simulink library "Custom_Library"  (R2023a)
settings: Solver=VariableStepAuto  StartTime=0.0  StopTime=10.0  RelTol=1e-3
values from neighbouring files (symbols this model uses):
  AEP = 0.03    [simulation_setup.m]
  max_torque_alpha = globalTorque    (= 0.94)    [simulation_setup.m]
  max_torque_beta = globalTorque    (= 0.94)    [simulation_setup.m]
  max_torque_gamma = globalTorque    (= 0.94)    [simulation_setup.m]
  N = 16    [rl_setup.m]
  PEP = -0.03    [simulation_setup.m]
  pid_D = 1    [simulation_setup.m]
  pid_filter_N = 1000    [simulation_setup.m]
  pid_I = 0.1    [simulation_setup.m]
  pid_P = 600    [simulation_setup.m]
  step_height = 0.06    [simulation_setup.m]
  step_length = 0.04    [simulation_setup.m]
undefined symbols (not defined in the file or in its folder): X, Y, Z
libraries: sm_lib x31, nesl_utility x13, $bdroot x5, slpidlib x3
(part 2 of 2)

== system Custom_Library/Hexapod Leg/Coxa ==
  Inertia : sm_lib/Body Elements/Inertia  InertiaType=Custom  Mass=0.02471  MassUnits=kg  CenterOfMass=[0, 0, 0]  CenterOfMassUnits=m  MomentsOfInertia=[2.154e-05, 2.657e-05, 2.925e-05]  MomentsOfInertiaUnits=kg*m^2  ProductsOfInertia=[-1.000000000000002e-11, -1.92741e-06, -1.22e-09]  ProductsOfInertiaUnits=kg*m^2  GraphicType=None  MarkerShape=Inertia  MarkerSize=20  GraphicVisPropType=SimpleVisualProperties  GraphicDiffuseColor=[0.5 0.5 0.5]  GraphicSpecularColor=[0.5 0.5 0.5 1.0]  GraphicAmbientColor=[0.15 0.15 0.15 1.0]  GraphicEmissiveColor=[0.0 0.0 0.0 1.0]  GraphicShininess=75  GraphicOpacity=1.0
  InertiaOriginTransform : sm_lib/Frames and Transforms/Rigid Transform  TranslationMethod=Cartesian  TranslationStandardOffset=0  TranslationStandardOffsetUnits=m  TranslationStandardAxis=+Z  TranslationCartesianOffset=[0.019066, -2e-06, 0.006577]  TranslationCartesianOffsetUnits=m  TranslationROffset=0  TranslationROffsetUnits=m  TranslationZOffset=0  TranslationZOffsetUnits=m  TranslationThetaOffset=0  TranslationThetaOffsetUnits=deg  RotationMethod=RotationSequence  RotationAngleUnits=deg  RotationStandardAxis=+Z  RotationAngle=0.0  RotationArbitraryAxis=[0 0 1]  FollAlignAxisA=+X  BaseAlignAxisA=+Y  FollAlignAxisB=+Y  BaseAlignAxisB=+Z  RotationSequenceAxes=BaseAxes  RotationSequence=XYZ  RotationSequenceAngles=[0, 0, 0]  RotationSequenceAnglesUnits=rad  RotationMatrix=[1 0 0; 0 1 0; 0 0 1]  Quaternion=[1 0 0 0]
  ReferenceFrame : sm_lib/Frames and Transforms/Reference Frame
  Spatial Contact Force : sm_lib/Forces and Torques/Spatial Contact Force  SenseContactBaseRotation=off  SenseContactBaseTranslation=off  CoefficientOfDynamicFriction=mu_dynamic  CoefficientOfStaticFriction=mu_static  NormalDamping=damping  NormalDampingUnits=N/(m/s)  SenseContactSignal=off  NormalStiffness=stiffness  NormalStiffnessUnits=N/m  FrictionalCriticalVelocity=critical_vel  FrictionalCriticalVelocityUnits=m/s  ZeroCrossDetectContactStartAndEnd=off  SenseContactFollowerRotation=off  SenseContactFollowerTranslation=off  FrictionType=SmoothStickSlip  SenseFrictionalForceMagnitude=off  SenseNormalForceMagnitude=off  NormalForceType=SmoothSpringDamper  SenseNormalVelocity=off  SenseSeparationDistance=off  SenseTangentialVelocity=off  NormalTransitionRegionWidth=transition_region  NormalTransitionRegionWidthUnits=m
  Visual : sm_lib/Body Elements/File Solid  ExtGeomFileName=C:\Users\basti\OneDrive\Dokumente\Eigene Dokumente\Bachelorarbeit\Bachelor-Thesis\MATLAB\robot_models\interbotix_xshexapod_descriptions\meshes\pxmark4_meshes\pxmark4_coxa_link.stl  UnitType=Custom  ExtGeomFileUnits=mm  StepReaderType=HEX  ExportConvexHullGeometry=on  InertiaType=Custom  Mass=0  MassUnits=kg  CenterOfMass=[0, 0, 0]  CenterOfMassUnits=m  MomentsOfInertia=[0, 0, 0]  MomentsOfInertiaUnits=kg*m^2  ProductsOfInertia=[0, 0, 0]  ProductsOfInertiaUnits=kg*m^2  BasedOnType=DensityFromFile  Density=1000  DensityUnits=kg/m^3  DoExposeReferenceFrame=on  SerializedFrames=<Frames/>  GraphicType=FromGeometry  MarkerShape=Sphere  MarkerSize=10  GraphicVisPropType=SimpleVisualProperties  GraphicDiffuseColor=[0.5, 0.5, 0.5]  GraphicSpecularColor=[0.5 0.5 0.5 1.0]  GraphicAmbientColor=[0.15 0.15 0.15 1.0]  GraphicEmissiveColor=[0.0 0.0 0.0 1.0]  GraphicShininess=75  GraphicOpacity=1
  VisualOriginTransform : sm_lib/Frames and Transforms/Rigid Transform  TranslationMethod=Cartesian  TranslationStandardOffset=0  TranslationStandardOffsetUnits=m  TranslationStandardAxis=+Z  TranslationCartesianOffset=[0, 0, 0]  TranslationCartesianOffsetUnits=m  TranslationROffset=0  TranslationROffsetUnits=m  TranslationZOffset=0  TranslationZOffsetUnits=m  TranslationThetaOffset=0  TranslationThetaOffsetUnits=deg  RotationMethod=RotationSequence  RotationAngleUnits=deg  RotationStandardAxis=+Z  RotationAngle=0.0  RotationArbitraryAxis=[0 0 1]  FollAlignAxisA=+X  BaseAlignAxisA=+Y  FollAlignAxisB=+Y  BaseAlignAxisB=+Z  RotationSequenceAxes=BaseAxes  RotationSequence=XYZ  RotationSequenceAngles=[0, 0, 0]  RotationSequenceAnglesUnits=rad  RotationMatrix=[1 0 0; 0 1 0; 0 0 1]  Quaternion=[1 0 0 0]
  left_front_coxa_AxisInvTransform : sm_lib/Frames and Transforms/Rigid Transform  TranslationMethod=Cartesian  TranslationStandardOffset=0  TranslationStandardOffsetUnits=m  TranslationStandardAxis=+Z  TranslationCartesianOffset=[0, 0, 0]  TranslationCartesianOffsetUnits=m  TranslationROffset=0  TranslationROffsetUnits=m  TranslationZOffset=0  TranslationZOffsetUnits=m  TranslationThetaOffset=0  TranslationThetaOffsetUnits=deg  RotationMethod=ArbitraryAxis  RotationAngleUnits=rad  RotationStandardAxis=+Z  RotationAngle=0  RotationArbitraryAxis=[1, 0, 0]  FollAlignAxisA=+X  BaseAlignAxisA=+Y  FollAlignAxisB=+Y  BaseAlignAxisB=+Z  RotationSequenceAxes=FollowerAxes  RotationSequence=XYX  RotationSequenceAngles=[0 0 0]  RotationSequenceAnglesUnits=deg  RotationMatrix=[1 0 0; 0 1 0; 0 0 1]  Quaternion=[1 0 0 0]
  left_front_femur_AxisTransform : sm_lib/Frames and Transforms/Rigid Transform  TranslationMethod=Cartesian  TranslationStandardOffset=0  TranslationStandardOffsetUnits=m  TranslationStandardAxis=+Z  TranslationCartesianOffset=[0, 0, 0]  TranslationCartesianOffsetUnits=m  TranslationROffset=0  TranslationROffsetUnits=m  TranslationZOffset=0  TranslationZOffsetUnits=m  TranslationThetaOffset=0  TranslationThetaOffsetUnits=deg  RotationMethod=ArbitraryAxis  RotationAngleUnits=rad  RotationStandardAxis=+Z  RotationAngle=1.570796326794897  RotationArbitraryAxis=[-1, 0, 0]  FollAlignAxisA=+X  BaseAlignAxisA=+Y  FollAlignAxisB=+Y  BaseAlignAxisB=+Z  RotationSequenceAxes=FollowerAxes  RotationSequence=XYX  RotationSequenceAngles=[0 0 0]  RotationSequenceAnglesUnits=deg  RotationMatrix=[1 0 0; 0 1 0; 0 0 1]  Quaternion=[1 0 0 0]
  left_front_femur_OriginTransform : sm_lib/Frames and Transforms/Rigid Transform  TranslationMethod=Cartesian  TranslationStandardOffset=0  TranslationStandardOffsetUnits=m  TranslationStandardAxis=+Z  TranslationCartesianOffset=[0.052907539, 0, 0]  TranslationCartesianOffsetUnits=m  TranslationROffset=0  TranslationROffsetUnits=m  TranslationZOffset=0  TranslationZOffsetUnits=m  TranslationThetaOffset=0  TranslationThetaOffsetUnits=deg  RotationMethod=RotationSequence  RotationAngleUnits=deg  RotationStandardAxis=+Z  RotationAngle=0.0  RotationArbitraryAxis=[0 0 1]  FollAlignAxisA=+X  BaseAlignAxisA=+Y  FollAlignAxisB=+Y  BaseAlignAxisB=+Z  RotationSequenceAxes=BaseAxes  RotationSequence=XYZ  RotationSequenceAngles=[0, 0, 0]  RotationSequenceAnglesUnits=rad  RotationMatrix=[1 0 0; 0 1 0; 0 0 1]  Quaternion=[1 0 0 0]
  F : PMIOPort  Side=Left
  G : PMIOPort  Port=2  Side=Left
  F1 : PMIOPort  Port=3  Side=Right
  connections:
  Inertia/RConn1 -- InertiaOriginTransform/RConn1
  ReferenceFrame/RConn1 -- InertiaOriginTransform/LConn1 -- left_front_coxa_AxisInvTransform/LConn1 -- left_front_femur_OriginTransform/LConn1 -- VisualOriginTransform/LConn1
  Visual/RConn1 -- VisualOriginTransform/RConn1
  left_front_coxa_AxisInvTransform/RConn1 -- F/RConn1
  left_front_femur_AxisTransform/RConn1 -- F1/RConn1
  left_front_femur_AxisTransform/LConn1 -- left_front_femur_OriginTransform/RConn1
  G/RConn1 -- Spatial Contact Force/LConn1
  Spatial Contact Force/RConn1 -- Visual/LConn1

== system Custom_Library/Hexapod Leg/Femur ==
  Inertia : sm_lib/Body Elements/Inertia  InertiaType=Custom  Mass=0.08583399999999999  MassUnits=kg  CenterOfMass=[0, 0, 0]  CenterOfMassUnits=m  MomentsOfInertia=[2.887e-05, 7.502e-05, 8.672e-05]  MomentsOfInertiaUnits=kg*m^2  ProductsOfInertia=[2.999999999999994e-10, 4.8494e-06, 2.419e-07]  ProductsOfInertiaUnits=kg*m^2  GraphicType=None  MarkerShape=Inertia  MarkerSize=20  GraphicVisPropType=SimpleVisualProperties  GraphicDiffuseColor=[0.5 0.5 0.5]  GraphicSpecularColor=[0.5 0.5 0.5 1.0]  GraphicAmbientColor=[0.15 0.15 0.15 1.0]  GraphicEmissiveColor=[0.0 0.0 0.0 1.0]  GraphicShininess=75  GraphicOpacity=1.0
  InertiaOriginTransform : sm_lib/Frames and Transforms/Rigid Transform  TranslationMethod=Cartesian  TranslationStandardOffset=0  TranslationStandardOffsetUnits=m  TranslationStandardAxis=+Z  TranslationCartesianOffset=[0.020226, -0.00029, -0.00063]  TranslationCartesianOffsetUnits=m  TranslationROffset=0  TranslationROffsetUnits=m  TranslationZOffset=0  TranslationZOffsetUnits=m  TranslationThetaOffset=0  TranslationThetaOffsetUnits=deg  RotationMethod=RotationSequence  RotationAngleUnits=deg  RotationStandardAxis=+Z  RotationAngle=0.0  RotationArbitraryAxis=[0 0 1]  FollAlignAxisA=+X  BaseAlignAxisA=+Y  FollAlignAxisB=+Y  BaseAlignAxisB=+Z  RotationSequenceAxes=BaseAxes  RotationSequence=XYZ  RotationSequenceAngles=[0, 0, 0]  RotationSequenceAnglesUnits=rad  RotationMatrix=[1 0 0; 0 1 0; 0 0 1]  Quaternion=[1 0 0 0]
  ReferenceFrame : sm_lib/Frames and Transforms/Reference Frame
  Spatial Contact Force : sm_lib/Forces and Torques/Spatial Contact Force  SenseContactBaseRotation=off  SenseContactBaseTranslation=off  CoefficientOfDynamicFriction=mu_dynamic  CoefficientOfStaticFriction=mu_static  NormalDamping=damping  NormalDampingUnits=N/(m/s)  SenseContactSignal=off  NormalStiffness=stiffness  NormalStiffnessUnits=N/m  FrictionalCriticalVelocity=critical_vel  FrictionalCriticalVelocityUnits=m/s  ZeroCrossDetectContactStartAndEnd=off  SenseContactFollowerRotation=off  SenseContactFollowerTranslation=off  FrictionType=SmoothStickSlip  SenseFrictionalForceMagnitude=off  SenseNormalForceMagnitude=off  NormalForceType=SmoothSpringDamper  SenseNormalVelocity=off  SenseSeparationDistance=off  SenseTangentialVelocity=off  NormalTransitionRegionWidth=transition_region  NormalTransitionRegionWidthUnits=m
  Visual : sm_lib/Body Elements/File Solid  ExtGeomFileName=C:\Users\basti\OneDrive\Dokumente\Eigene Dokumente\Bachelorarbeit\Bachelor-Thesis\MATLAB\robot_models\interbotix_xshexapod_descriptions\meshes\pxmark4_meshes\pxmark4_femur_link.stl  UnitType=Custom  ExtGeomFileUnits=mm  StepReaderType=HEX  ExportConvexHullGeometry=on  InertiaType=Custom  Mass=0  MassUnits=kg  CenterOfMass=[0, 0, 0]  CenterOfMassUnits=m  MomentsOfInertia=[0, 0, 0]  MomentsOfInertiaUnits=kg*m^2  ProductsOfInertia=[0, 0, 0]  ProductsOfInertiaUnits=kg*m^2  BasedOnType=DensityFromFile  Density=1000  DensityUnits=kg/m^3  DoExposeReferenceFrame=on  SerializedFrames=<Frames/>  GraphicType=FromGeometry  MarkerShape=Sphere  MarkerSize=10  GraphicVisPropType=SimpleVisualProperties  GraphicDiffuseColor=[0.5, 0.5, 0.5]  GraphicSpecularColor=[0.5 0.5 0.5 1.0]  GraphicAmbientColor=[0.15 0.15 0.15 1.0]  GraphicEmissiveColor=[0.0 0.0 0.0 1.0]  GraphicShininess=75  GraphicOpacity=1
  VisualOriginTransform : sm_lib/Frames and Transforms/Rigid Transform  TranslationMethod=Cartesian  TranslationStandardOffset=0  TranslationStandardOffsetUnits=m  TranslationStandardAxis=+Z  TranslationCartesianOffset=[0, 0, 0]  TranslationCartesianOffsetUnits=m  TranslationROffset=0  TranslationROffsetUnits=m  TranslationZOffset=0  TranslationZOffsetUnits=m  TranslationThetaOffset=0  TranslationThetaOffsetUnits=deg  RotationMethod=RotationSequence  RotationAngleUnits=deg  RotationStandardAxis=+Z  RotationAngle=0.0  RotationArbitraryAxis=[0 0 1]  FollAlignAxisA=+X  BaseAlignAxisA=+Y  FollAlignAxisB=+Y  BaseAlignAxisB=+Z  RotationSequenceAxes=BaseAxes  RotationSequence=XYZ  RotationSequenceAngles=[0, 0, 0]  RotationSequenceAnglesUnits=rad  RotationMatrix=[1 0 0; 0 1 0; 0 0 1]  Quaternion=[1 0 0 0]
  left_front_femur_AxisInvTransform : sm_lib/Frames and Transforms/Rigid Transform  TranslationMethod=Cartesian  TranslationStandardOffset=0  TranslationStandardOffsetUnits=m  TranslationStandardAxis=+Z  TranslationCartesianOffset=[0, 0, 0]  TranslationCartesianOffsetUnits=m  TranslationROffset=0  TranslationROffsetUnits=m  TranslationZOffset=0  TranslationZOffsetUnits=m  TranslationThetaOffset=0  TranslationThetaOffsetUnits=deg  RotationMethod=ArbitraryAxis  RotationAngleUnits=rad  RotationStandardAxis=+Z  RotationAngle=1.570796326794897  RotationArbitraryAxis=[-1, 0, 0]  FollAlignAxisA=+X  BaseAlignAxisA=+Y  FollAlignAxisB=+Y  BaseAlignAxisB=+Z  RotationSequenceAxes=FollowerAxes  RotationSequence=XYX  RotationSequenceAngles=[0 0 0]  RotationSequenceAnglesUnits=deg  RotationMatrix=[1 0 0; 0 1 0; 0 0 1]  Quaternion=[1 0 0 0]
  left_front_tibia_AxisTransform : sm_lib/Frames and Transforms/Rigid Transform  TranslationMethod=Cartesian  TranslationStandardOffset=0  TranslationStandardOffsetUnits=m  TranslationStandardAxis=+Z  TranslationCartesianOffset=[0, 0, 0]  TranslationCartesianOffsetUnits=m  TranslationROffset=0  TranslationROffsetUnits=m  TranslationZOffset=0  TranslationZOffsetUnits=m  TranslationThetaOffset=0  TranslationThetaOffsetUnits=deg  RotationMethod=ArbitraryAxis  RotationAngleUnits=rad  RotationStandardAxis=+Z  RotationAngle=1.570796326794897  RotationArbitraryAxis=[-1, 0, 0]  FollAlignAxisA=+X  BaseAlignAxisA=+Y  FollAlignAxisB=+Y  BaseAlignAxisB=+Z  RotationSequenceAxes=FollowerAxes  RotationSequence=XYX  RotationSequenceAngles=[0 0 0]  RotationSequenceAnglesUnits=deg  RotationMatrix=[1 0 0; 0 1 0; 0 0 1]  Quaternion=[1 0 0 0]
  left_front_tibia_OriginTransform : sm_lib/Frames and Transforms/Rigid Transform  TranslationMethod=Cartesian  TranslationStandardOffset=0  TranslationStandardOffsetUnits=m  TranslationStandardAxis=+Z  TranslationCartesianOffset=[0.06, 0, -0.015]  TranslationCartesianOffsetUnits=m  TranslationROffset=0  TranslationROffsetUnits=m  TranslationZOffset=0  TranslationZOffsetUnits=m  TranslationThetaOffset=0  TranslationThetaOffsetUnits=deg  RotationMethod=RotationSequence  RotationAngleUnits=deg  RotationStandardAxis=+Z  RotationAngle=0.0  RotationArbitraryAxis=[0 0 1]  FollAlignAxisA=+X  BaseAlignAxisA=+Y  FollAlignAxisB=+Y  BaseAlignAxisB=+Z  RotationSequenceAxes=BaseAxes  RotationSequence=XYZ  RotationSequenceAngles=[0, 0, 0]  RotationSequenceAnglesUnits=rad  RotationMatrix=[1 0 0; 0 1 0; 0 0 1]  Quaternion=[1 0 0 0]
  F : PMIOPort  Side=Left
  G : PMIOPort  Port=2  Side=Left
  F1 : PMIOPort  Port=3  Side=Right
  connections:
  Inertia/RConn1 -- InertiaOriginTransform/RConn1
  ReferenceFrame/RConn1 -- InertiaOriginTransform/LConn1 -- left_front_femur_AxisInvTransform/LConn1 -- left_front_tibia_OriginTransform/LConn1 -- VisualOriginTransform/LConn1
  Visual/RConn1 -- VisualOriginTransform/RConn1
  left_front_femur_AxisInvTransform/RConn1 -- F/RConn1
  left_front_tibia_AxisTransform/RConn1 -- F1/RConn1
  left_front_tibia_AxisTransform/LConn1 -- left_front_tibia_OriginTransform/RConn1
  Spatial Contact Force/RConn1 -- Visual/LConn1
  G/RConn1 -- Spatial Contact Force/LConn1

== system Custom_Library/Hexapod Leg/Tibia ==
  Inertia : sm_lib/Body Elements/Inertia  InertiaType=Custom  Mass=0.171825  MassUnits=kg  CenterOfMass=[0, 0, 0]  CenterOfMassUnits=m  MomentsOfInertia=[0.0001762, 0.0005158, 0.0003768000000000001]  MomentsOfInertiaUnits=kg*m^2  ProductsOfInertia=[6.181e-07, 0.0001789, -1.4522e-06]  ProductsOfInertiaUnits=kg*m^2  GraphicType=None  MarkerShape=Inertia  MarkerSize=20  GraphicVisPropType=SimpleVisualProperties  GraphicDiffuseColor=[0.5 0.5 0.5]  GraphicSpecularColor=[0.5 0.5 0.5 1.0]  GraphicAmbientColor=[0.15 0.15 0.15 1.0]  GraphicEmissiveColor=[0.0 0.0 0.0 1.0]  GraphicShininess=75  GraphicOpacity=1.0
  InertiaOriginTransform : sm_lib/Frames and Transforms/Rigid Transform  TranslationMethod=Cartesian  TranslationStandardOffset=0  TranslationStandardOffsetUnits=m  TranslationStandardAxis=+Z  TranslationCartesianOffset=[0.036797, 5.4e-05, -0.011991]  TranslationCartesianOffsetUnits=m  TranslationROffset=0  TranslationROffsetUnits=m  TranslationZOffset=0  TranslationZOffsetUnits=m  TranslationThetaOffset=0  TranslationThetaOffsetUnits=deg  RotationMethod=RotationSequence  RotationAngleUnits=deg  RotationStandardAxis=+Z  RotationAngle=0.0  RotationArbitraryAxis=[0 0 1]  FollAlignAxisA=+X  BaseAlignAxisA=+Y  FollAlignAxisB=+Y  BaseAlignAxisB=+Z  RotationSequenceAxes=BaseAxes  RotationSequence=XYZ  RotationSequenceAngles=[0, 0, 0]  RotationSequenceAnglesUnits=rad  RotationMatrix=[1 0 0; 0 1 0; 0 0 1]  Quaternion=[1 0 0 0]
  ReferenceFrame : sm_lib/Frames and Transforms/Reference Frame
  Spatial Contact Force : sm_lib/Forces and Torques/Spatial Contact Force  SenseContactBaseRotation=off  SenseContactBaseTranslation=off  CoefficientOfDynamicFriction=mu_dynamic  CoefficientOfStaticFriction=mu_static  NormalDamping=damping  NormalDampingUnits=N/(m/s)  SenseContactSignal=off  NormalStiffness=stiffness  NormalStiffnessUnits=N/m  FrictionalCriticalVelocity=critical_vel  FrictionalCriticalVelocityUnits=m/s  ZeroCrossDetectContactStartAndEnd=off  SenseContactFollowerRotation=off  SenseContactFollowerTranslation=off  FrictionType=SmoothStickSlip  SenseFrictionalForceMagnitude=off  SenseNormalForceMagnitude=off  NormalForceType=SmoothSpringDamper  SenseNormalVelocity=off  SenseSeparationDistance=off  SenseTangentialVelocity=off  NormalTransitionRegionWidth=transition_region  NormalTransitionRegionWidthUnits=m
  Visual : sm_lib/Body Elements/File Solid  ExtGeomFileName=C:\Users\basti\OneDrive\Dokumente\Eigene Dokumente\Bachelorarbeit\Bachelor-Thesis\MATLAB\robot_models\interbotix_xshexapod_descriptions\meshes\pxmark4_meshes\pxmark4_tibia_link.stl  UnitType=Custom  ExtGeomFileUnits=mm  StepReaderType=HEX  ExportConvexHullGeometry=on  InertiaType=Custom  Mass=0  MassUnits=kg  CenterOfMass=[0, 0, 0]  CenterOfMassUnits=m  MomentsOfInertia=[0, 0, 0]  MomentsOfInertiaUnits=kg*m^2  ProductsOfInertia=[0, 0, 0]  ProductsOfInertiaUnits=kg*m^2  BasedOnType=DensityFromFile  Density=1000  DensityUnits=kg/m^3  DoExposeReferenceFrame=on  SerializedFrames=<Frames/>  GraphicType=FromGeometry  MarkerShape=Sphere  MarkerSize=10  GraphicVisPropType=SimpleVisualProperties  GraphicDiffuseColor=[0.5, 0.5, 0.5]  GraphicSpecularColor=[0.5 0.5 0.5 1.0]  GraphicAmbientColor=[0.15 0.15 0.15 1.0]  GraphicEmissiveColor=[0.0 0.0 0.0 1.0]  GraphicShininess=75  GraphicOpacity=1
  VisualOriginTransform : sm_lib/Frames and Transforms/Rigid Transform  TranslationMethod=Cartesian  TranslationStandardOffset=0  TranslationStandardOffsetUnits=m  TranslationStandardAxis=+Z  TranslationCartesianOffset=[0, 0, 0]  TranslationCartesianOffsetUnits=m  TranslationROffset=0  TranslationROffsetUnits=m  TranslationZOffset=0  TranslationZOffsetUnits=m  TranslationThetaOffset=0  TranslationThetaOffsetUnits=deg  RotationMethod=RotationSequence  RotationAngleUnits=deg  RotationStandardAxis=+Z  RotationAngle=0.0  RotationArbitraryAxis=[0 0 1]  FollAlignAxisA=+X  BaseAlignAxisA=+Y  FollAlignAxisB=+Y  BaseAlignAxisB=+Z  RotationSequenceAxes=BaseAxes  RotationSequence=XYZ  RotationSequenceAngles=[0, 0, 0]  RotationSequenceAnglesUnits=rad  RotationMatrix=[1 0 0; 0 1 0; 0 0 1]  Quaternion=[1 0 0 0]
  left_front_foot_OriginTransform : sm_lib/Frames and Transforms/Rigid Transform  TranslationMethod=Cartesian  TranslationStandardOffset=0  TranslationStandardOffsetUnits=m  TranslationStandardAxis=+Z  TranslationCartesianOffset=[0.095, 0, -0.09]  TranslationCartesianOffsetUnits=m  TranslationROffset=0  TranslationROffsetUnits=m  TranslationZOffset=0  TranslationZOffsetUnits=m  TranslationThetaOffset=0  TranslationThetaOffsetUnits=deg  RotationMethod=RotationSequence  RotationAngleUnits=deg  RotationStandardAxis=+Z  RotationAngle=0.0  RotationArbitraryAxis=[0 0 1]  FollAlignAxisA=+X  BaseAlignAxisA=+Y  FollAlignAxisB=+Y  BaseAlignAxisB=+Z  RotationSequenceAxes=BaseAxes  RotationSequence=XYZ  RotationSequenceAngles=[0, 0, 0]  RotationSequenceAnglesUnits=rad  RotationMatrix=[1 0 0; 0 1 0; 0 0 1]  Quaternion=[1 0 0 0]
  left_front_tibia_AxisInvTransform : sm_lib/Frames and Transforms/Rigid Transform  TranslationMethod=Cartesian  TranslationStandardOffset=0  TranslationStandardOffsetUnits=m  TranslationStandardAxis=+Z  TranslationCartesianOffset=[0, 0, 0]  TranslationCartesianOffsetUnits=m  TranslationROffset=0  TranslationROffsetUnits=m  TranslationZOffset=0  TranslationZOffsetUnits=m  TranslationThetaOffset=0  TranslationThetaOffsetUnits=deg  RotationMethod=ArbitraryAxis  RotationAngleUnits=rad  RotationStandardAxis=+Z  RotationAngle=1.570796326794897  RotationArbitraryAxis=[-1, 0, 0]  FollAlignAxisA=+X  BaseAlignAxisA=+Y  FollAlignAxisB=+Y  BaseAlignAxisB=+Z  RotationSequenceAxes=FollowerAxes  RotationSequence=XYX  RotationSequenceAngles=[0 0 0]  RotationSequenceAnglesUnits=deg  RotationMatrix=[1 0 0; 0 1 0; 0 0 1]  Quaternion=[1 0 0 0]
  F : PMIOPort  Side=Left
  G : PMIOPort  Port=2  Side=Left
  F1 : PMIOPort  Port=3  Side=Right
  connections:
  Inertia/RConn1 -- InertiaOriginTransform/RConn1
  ReferenceFrame/RConn1 -- InertiaOriginTransform/LConn1 -- left_front_foot_OriginTransform/LConn1 -- left_front_tibia_AxisInvTransform/LConn1 -- VisualOriginTransform/LConn1
  Visual/RConn1 -- VisualOriginTransform/RConn1
  left_front_foot_OriginTransform/RConn1 -- F1/RConn1
  left_front_tibia_AxisInvTransform/RConn1 -- F/RConn1
  Spatial Contact Force/RConn1 -- Visual/LConn1
  G/RConn1 -- Spatial Contact Force/LConn1

== system Custom_Library/Hexapod Leg/Torque Limiting ==
  Input : Inport
  Alpha Limit : Saturate  UpperLimit=max_torque_alpha  LowerLimit=-max_torque_alpha
  Beta Limit : Saturate  UpperLimit=max_torque_beta  LowerLimit=-max_torque_beta
  Bus Selector1 : BusSelector  OutputSignals=torque_alpha,torque_beta,torque_gamma
  Gamma Limit : Saturate  UpperLimit=max_torque_gamma  LowerLimit=-max_torque_gamma
  Alpha : Outport
  Beta : Outport  Port=2
  Gamma : Outport  Port=3
  wires:
  Bus Selector1/1 -> Alpha Limit/1  "<torque_alpha>"
  Input/1 -> Bus Selector1/1
  Bus Selector1/3 -> Gamma Limit/1  "<torque_gamma>"
  Bus Selector1/2 -> Beta Limit/1  "<torque_beta>"
  Alpha Limit/1 -> Alpha/1
  Beta Limit/1 -> Beta/1
  Gamma Limit/1 -> Gamma/1

== system Custom_Library/Signal Generator Linear X (Gen. 2)/Stance Phase ==
  Frequency : Inport
  Reset : ResetPort  DisableCoverage=on
  Add : Sum
  Constant1 : Constant  Value=x_amplitude
  Constant2 : Constant  Value=0
  Constant5 : Constant  Value=x_amplitude
  Constant6 : Constant
  Gain1 : Gain  Gain=-4
  Integrator1 : Integrator
  Product2 : Product
  Product3 : Product
  Saturation : Saturate  UpperLimit=step_length  LowerLimit=-step_length
  X : Outport
  "Z " : Outport  Port=2
  wires:
  Constant2/1 -> "Z "/1
  Constant5/1 -> Add/1
  Constant6/1 -> Integrator1/1
  Add/1 -> Saturation/1
  Product3/1 -> Add/2
  Integrator1/1 -> Product3/2
  Frequency/1 -> Product2/2
  Gain1/1 -> Product2/1
  Product2/1 -> Product3/1
  Saturation/1 -> X/1
  Constant1/1 -> Gain1/1

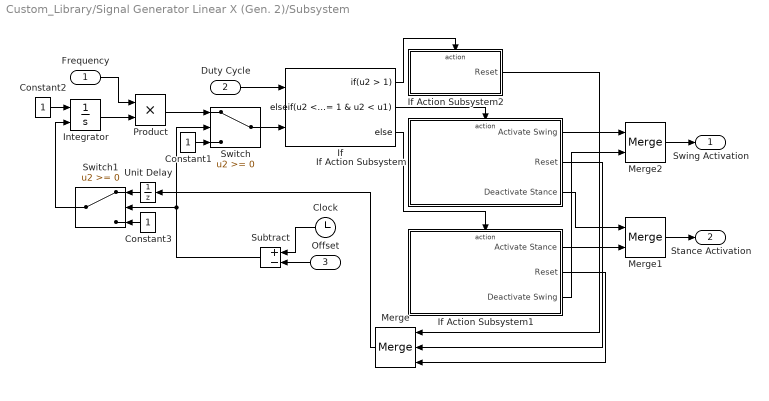
== system Custom_Library/Signal Generator Linear X (Gen. 2)/Subsystem ==
  Frequency : Inport
  Duty Cycle : Inport  Port=2
  Offset : Inport  Port=3
  Clock : Clock
  Constant1 : Constant
  Constant2 : Constant
  Constant3 : Constant
  If : If  NumInputs=2  IfExpression=u2 > 1  ElseIfExpressions=u2 <= 1 & u2 < u1
  If Action Subsystem : Subsystem  TreatAsAtomicUnit=on
  If Action Subsystem1 : Subsystem  TreatAsAtomicUnit=on
  If Action Subsystem2 : Subsystem  TreatAsAtomicUnit=on
  Integrator : Integrator  ExternalReset=level
  Merge : Merge  Inputs=3
  Merge1 : Merge
  Merge2 : Merge
  Product : Product
  Subtract : Sum  Inputs=+-
  Switch : Switch  SaturateOnIntegerOverflow=off  InputSameDT=off
  Switch1 : Switch  SaturateOnIntegerOverflow=off  InputSameDT=off
  Unit Delay : UnitDelay  SampleTime=-1  HasFrameUpgradeWarning=on
  Swing Activation : Outport
  Stance Activation : Outport  Port=2
  wires:
  If Action Subsystem/3(Deactivate Stance) -> Merge1/1
  If/2 -> If Action Subsystem/Action
  Duty Cycle/1 -> If/1
  If/1 -> If Action Subsystem2/Action
  If Action Subsystem1/1(Activate Stance) -> Merge1/2
  If Action Subsystem/2(Reset) -> Merge/2
  Merge/1 -> Unit Delay/1
  If Action Subsystem1/3(Deactivate Swing) -> Merge2/2
  If Action Subsystem2/1(Reset) -> Merge/1
  If Action Subsystem/1(Activate Swing) -> Merge2/1
  If Action Subsystem1/2(Reset) -> Merge/3
  If/3 -> If Action Subsystem1/Action
  Merge2/1 -> Swing Activation/1
  Merge1/1 -> Stance Activation/1
  Switch/1 -> If/2
  Constant1/1 -> Switch/3
  Subtract/1 -> Switch1/2, Switch/2
  Offset/1 -> Subtract/2
  Clock/1 -> Subtract/1
  Integrator/1 -> Product/2
  Product/1 -> Switch/1
  Frequency/1 -> Product/1
  Constant2/1 -> Integrator/1
  Unit Delay/1 -> Switch1/1
  Constant3/1 -> Switch1/3
  Switch1/1 -> Integrator/2

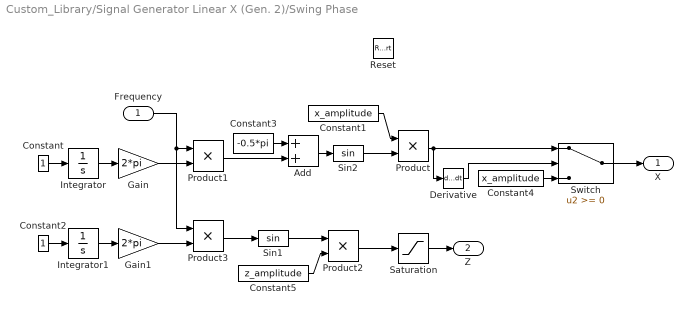
== system Custom_Library/Signal Generator Linear X (Gen. 2)/Swing Phase ==
  Frequency : Inport
  Reset : ResetPort  DisableCoverage=on
  Add : Sum
  Constant : Constant
  Constant1 : Constant  Value=x_amplitude
  Constant2 : Constant
  Constant3 : Constant  Value=-0.5*pi
  Constant4 : Constant  Value=x_amplitude
  Constant5 : Constant  Value=z_amplitude
  Derivative : Derivative
  Gain : Gain  Gain=2*pi
  Gain1 : Gain  Gain=2*pi
  Integrator : Integrator
  Integrator1 : Integrator
  Product{,1..3} (4 alike) : Product
  Saturation : Saturate  UpperLimit=step_height  LowerLimit=0
  Sin1 : Trigonometry
  Sin2 : Trigonometry
  Switch : Switch  SaturateOnIntegerOverflow=off  InputSameDT=off
  X : Outport
  "Z " : Outport  Port=2
  wires:
  Integrator/1 -> Gain/1
  Constant/1 -> Integrator/1
  Sin2/1 -> Product/2
  Constant1/1 -> Product/1
  Product2/1 -> Saturation/1
  Gain/1 -> Product1/2
  Add/1 -> Sin2/1
  Product1/1 -> Add/2
  Constant3/1 -> Add/1
  Product/1 -> Switch/1, Derivative/1
  Constant4/1 -> Switch/3
  Switch/1 -> X/1
  Derivative/1 -> Switch/2
  Product3/1 -> Sin1/1
  Sin1/1 -> Product2/1
  Constant5/1 -> Product2/2
  Constant2/1 -> Integrator1/1
  Gain1/1 -> Product3/2
  Integrator1/1 -> Gain1/1
  Frequency/1 -> Product3/1, Product1/1
  Saturation/1 -> "Z "/1

== system Custom_Library/Signal Generator(Gen. 2)/Stance Phase ==
  Frequency : Inport
  Reset : ResetPort  DisableCoverage=on
  Add : Sum
  Constant : Constant
  Constant1 : Constant  Value=step_length
  Constant2 : Constant  Value=0
  Constant3 : Constant  Value=0.5*pi
  Constant4 : Constant  Value=-step_length
  Derivative : Derivative
  Gain : Gain  Gain=2*pi
  Integrator : Integrator
  Product : Product
  Product1 : Product
  Sin : Trigonometry
  Switch : Switch  Criteria=u2 > Threshold  SaturateOnIntegerOverflow=off  InputSameDT=off
  X : Outport
  "Z " : Outport  Port=2
  wires:
  Integrator/1 -> Gain/1
  Constant/1 -> Integrator/1
  Sin/1 -> Product/2
  Constant1/1 -> Product/1
  Constant2/1 -> "Z "/1
  Frequency/1 -> Product1/1
  Gain/1 -> Product1/2
  Add/1 -> Sin/1
  Product1/1 -> Add/2
  Constant3/1 -> Add/1
  Product/1 -> Derivative/1, Switch/3
  Switch/1 -> X/1
  Derivative/1 -> Switch/2
  Constant4/1 -> Switch/1

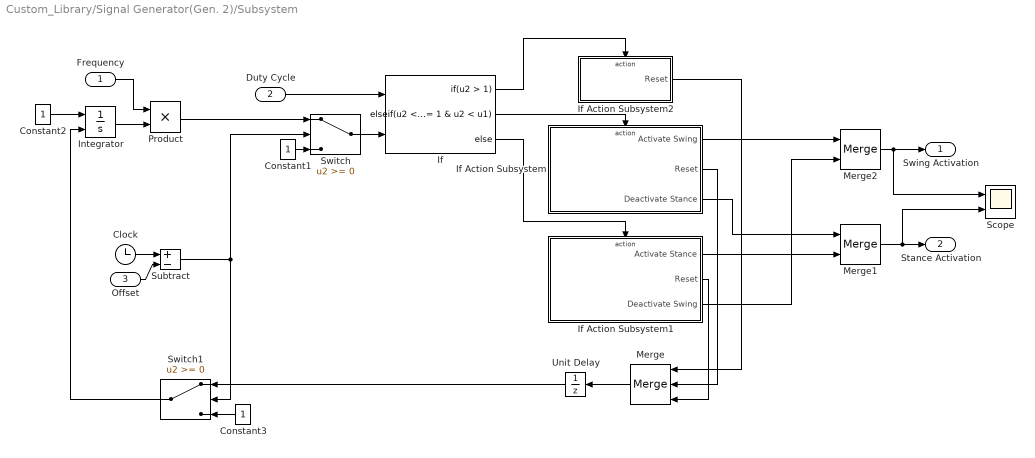
== system Custom_Library/Signal Generator(Gen. 2)/Subsystem ==
  Frequency : Inport
  Duty Cycle : Inport  Port=2
  Offset : Inport  Port=3
  Clock : Clock
  Constant1 : Constant
  Constant2 : Constant
  Constant3 : Constant
  If : If  NumInputs=2  IfExpression=u2 > 1  ElseIfExpressions=u2 <= 1 & u2 < u1
  If Action Subsystem : Subsystem  TreatAsAtomicUnit=on
  If Action Subsystem1 : Subsystem  TreatAsAtomicUnit=on
  If Action Subsystem2 : Subsystem  TreatAsAtomicUnit=on
  Integrator : Integrator  ExternalReset=level
  Merge : Merge  Inputs=3
  Merge1 : Merge
  Merge2 : Merge
  Product : Product
  Scope : Scope  NumInputPorts=2
  Subtract : Sum  Inputs=+-
  Switch : Switch  SaturateOnIntegerOverflow=off  InputSameDT=off
  Switch1 : Switch  SaturateOnIntegerOverflow=off  InputSameDT=off
  Unit Delay : UnitDelay  SampleTime=-1  HasFrameUpgradeWarning=on
  Swing Activation : Outport
  Stance Activation : Outport  Port=2
  wires:
  If Action Subsystem/3(Deactivate Stance) -> Merge1/1
  If/2 -> If Action Subsystem/Action
  Duty Cycle/1 -> If/1
  If/1 -> If Action Subsystem2/Action
  If Action Subsystem1/1(Activate Stance) -> Merge1/2
  If Action Subsystem/2(Reset) -> Merge/2
  Merge/1 -> Unit Delay/1
  If Action Subsystem1/3(Deactivate Swing) -> Merge2/2
  If Action Subsystem2/1(Reset) -> Merge/1
  If Action Subsystem/1(Activate Swing) -> Merge2/1
  If Action Subsystem1/2(Reset) -> Merge/3
  If/3 -> If Action Subsystem1/Action
  Merge2/1 -> Scope/1, Swing Activation/1
  Merge1/1 -> Scope/2, Stance Activation/1
  Switch/1 -> If/2
  Constant1/1 -> Switch/3
  Subtract/1 -> Switch1/2, Switch/2
  Offset/1 -> Subtract/2
  Clock/1 -> Subtract/1
  Integrator/1 -> Product/2
  Product/1 -> Switch/1
  Frequency/1 -> Product/1
  Constant2/1 -> Integrator/1
  Unit Delay/1 -> Switch1/1
  Constant3/1 -> Switch1/3
  Switch1/1 -> Integrator/2

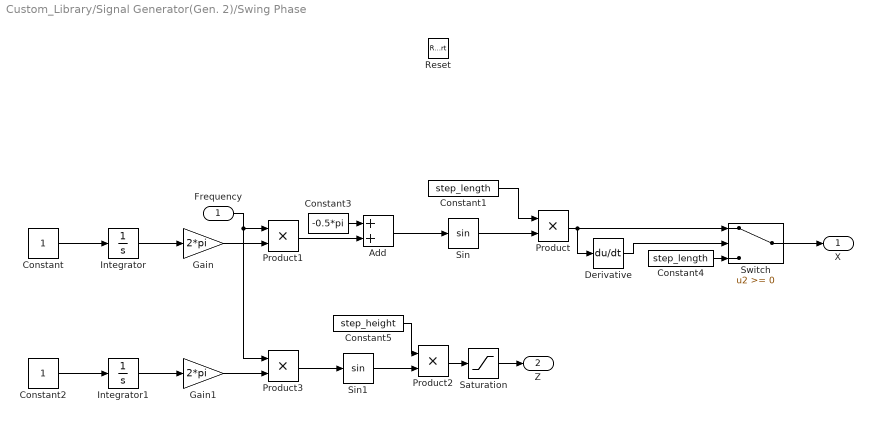
== system Custom_Library/Signal Generator(Gen. 2)/Swing Phase ==
  Frequency : Inport
  Reset : ResetPort  DisableCoverage=on
  Add : Sum
  Constant : Constant
  Constant1 : Constant  Value=step_length
  Constant2 : Constant
  Constant3 : Constant  Value=-0.5*pi
  Constant4 : Constant  Value=step_length
  Constant5 : Constant  Value=step_height
  Derivative : Derivative
  Gain : Gain  Gain=2*pi
  Gain1 : Gain  Gain=2*pi
  Integrator : Integrator
  Integrator1 : Integrator
  Product{,1..3} (4 alike) : Product
  Saturation : Saturate  UpperLimit=step_height  LowerLimit=0
  Sin : Trigonometry
  Sin1 : Trigonometry
  Switch : Switch  SaturateOnIntegerOverflow=off  InputSameDT=off
  X : Outport
  "Z " : Outport  Port=2
  wires:
  Integrator/1 -> Gain/1
  Constant/1 -> Integrator/1
  Sin/1 -> Product/2
  Constant1/1 -> Product/1
  Product2/1 -> Saturation/1
  Gain/1 -> Product1/2
  Add/1 -> Sin/1
  Product1/1 -> Add/2
  Constant3/1 -> Add/1
  Product/1 -> Switch/1, Derivative/1
  Constant4/1 -> Switch/3
  Switch/1 -> X/1
  Derivative/1 -> Switch/2
  Product3/1 -> Sin1/1
  Sin1/1 -> Product2/2
  Constant5/1 -> Product2/1
  Constant2/1 -> Integrator1/1
  Gain1/1 -> Product3/2
  Integrator1/1 -> Gain1/1
  Frequency/1 -> Product3/1, Product1/1
  Saturation/1 -> "Z "/1

== system Custom_Library/Swing-Stance Pattern Generation/Determine Frequencies ==
  note: (1/Hz) *duty_cycle = duty_cycle/Hz = swing_time
      |
      | 1/swing_time = 1 / (duty_cycle/Hz) = Hz/duty_cycle = Hz_for_swing
      | ----------------------------------------------------------------------------------------------------
      | (1/Hz)*(1-duty_cycle) = (1-duty_cycle)/Hz = stance_time
      |
      | 1/stance_time = 1 / ((1-duty_cycle)/Hz) = Hz / (1-duty_cycle) = Hz_for_stance
  Cycle Frequency [Hz] : Inport
  Duty Cycle [%] : Inport  Port=2
  Constant : Constant
  Divide : Product  Inputs=*/
  Divide1 : Product  Inputs=*/
  Subtract : Sum  Inputs=-+
  Swing Frequency [Hz] : Outport
  Stance Frequency [Hz] : Outport  Port=2
  wires:
  Constant/1 -> Subtract/2
  Subtract/1 -> Divide1/2
  Divide1/1 -> Stance Frequency [Hz]/1
  Cycle Frequency [Hz]/1 -> Divide/1, Divide1/1
  Duty Cycle [%]/1 -> Divide/2, Subtract/1
  Divide/1 -> Swing Frequency [Hz]/1

== system Custom_Library/Swing-Stance Pattern Generation/Swing-Stance Signal Generation ==
  note: Initiation of first Swing
      | enables the systems outputs.
      | Prevents stumbling.
  Swing Frequency [Hz] : Inport
  Stance Frequency [Hz] : Inport  Port=2
  Initiate Swing : Inport  Port=3
  Demux : Demux  Outputs=2
  Enable Outputs : Subsystem  TreatAsAtomicUnit=on
      settings: PortSchema="{\"entries\":[{\"content\":{\"sides\":[{\"content\":{\"connectorIds\":[\"In1\",\"In2\"]},\"type\":\"ConnectorPlacement.EquallySpacedRectSide\",\"uuid\":\"87b33ceb-5119-42f0-ab9e-44a74532733d\"},{\"content\":{\"connectorIds\":[\"Out1\",\"Out2\"],\"side\":\"RIGHT\"},\"type\":\"ConnectorPlacement.EquallySpacedRectSide\",\"uuid\":\"2748c539-b9f3-4627-a92c-05139a6ac450\"},{\"content\":{\"connectorIds\":[\"In3\"],\"side\":\"TOP\"},\"type\":\"ConnectorPlacement.EquallySpacedRectSide\",\"uuid\":\"98271061-2ac6-4173-8399-340c777b7c0e\"}]},\"type\":\"ConnectorPlacement.EquallySpacedConnector\",\"uuid\":\"a1ce645b-bfd3-4385-aaad-491949d96666\"}],\"packageUris\":[\"http://schema.mathworks.com/mf0/Connector/R2020b\"],\"version\":\"1.0\"}"
  Mux : Mux  Inputs=2
  Mux1 : Mux  Inputs=2
  NOT : Logic  Operator=NOT  IconShape=distinctive  AllPortsSameDT=off  OutDataTypeStr=boolean
  Switch1 : Switch  Criteria=u2 > Threshold  SaturateOnIntegerOverflow=off  InputSameDT=off
  Trajectory Generation - Stance Phase (Adaptive PEP) : Subsystem  TreatAsAtomicUnit=on
  Trajectory Generation - Swing Phase (Adaptive PEP) : Subsystem  TreatAsAtomicUnit=on
  Unit Delay : UnitDelay  SampleTime=-1  HasFrameUpgradeWarning=on
  X : Outport
  Z : Outport  Port=2
  wires:
  Enable Outputs/1(X out) -> X/1
  Enable Outputs/2(Z out) -> Z/1
  Switch1/1 -> Demux/1
  Demux/1 -> Enable Outputs/1(X in), Unit Delay/1
  Unit Delay/1 -> Trajectory Generation - Swing Phase (Adaptive PEP)/1(Leg X-Position)
  Stance Frequency [Hz]/1 -> Trajectory Generation - Stance Phase (Adaptive PEP)/1(Stance Frequency)
  Trajectory Generation - Stance Phase (Adaptive PEP)/2(Z) -> Mux/2
  Trajectory Generation - Swing Phase (Adaptive PEP)/2(Z) -> Mux1/2
  Trajectory Generation - Stance Phase (Adaptive PEP)/1(X) -> Mux/1
  Mux1/1 -> Switch1/1
  Trajectory Generation - Swing Phase (Adaptive PEP)/1(X) -> Mux1/1
  Demux/2 -> Enable Outputs/2(Z in)
  Mux/1 -> Switch1/3
  Initiate Swing/1 -> Enable Outputs/3(Enable), Trajectory Generation - Swing Phase (Adaptive PEP)/Reset
  NOT/1 -> Switch1/2
  Trajectory Generation - Swing Phase (Adaptive PEP)/3(Swing finished) -> NOT/1, Trajectory Generation - Stance Phase (Adaptive PEP)/Reset
  Swing Frequency [Hz]/1 -> Trajectory Generation - Swing Phase (Adaptive PEP)/2(Swing Frequency)

== system Custom_Library/Signal Generator Linear X (Gen. 2)/Subsystem/If Action Subsystem ==
  Action Port : ActionPort
  Constant : Constant
  Constant1 : Constant  Value=0
  Constant2 : Constant  Value=0
  Activate Swing : Outport
  Reset : Outport  Port=2
  Deactivate Stance : Outport  Port=3
  wires:
  Constant/1 -> Activate Swing/1
  Constant1/1 -> Reset/1
  Constant2/1 -> Deactivate Stance/1

== system Custom_Library/Signal Generator Linear X (Gen. 2)/Subsystem/If Action Subsystem1 ==
  Action Port : ActionPort
  Constant : Constant
  Constant1 : Constant  Value=0
  Constant2 : Constant  Value=0
  Activate Stance : Outport
  Reset : Outport  Port=2
  Deactivate Swing : Outport  Port=3
  wires:
  Constant/1 -> Activate Stance/1
  Constant1/1 -> Reset/1
  Constant2/1 -> Deactivate Swing/1

== system Custom_Library/Signal Generator Linear X (Gen. 2)/Subsystem/If Action Subsystem2 ==
  Action Port : ActionPort
  Constant1 : Constant
  Reset : Outport
  wires:
  Constant1/1 -> Reset/1

== system Custom_Library/Signal Generator(Gen. 2)/Subsystem/If Action Subsystem ==
  Action Port : ActionPort
  Constant : Constant
  Constant1 : Constant  Value=0
  Constant2 : Constant  Value=0
  Activate Swing : Outport
  Reset : Outport  Port=2
  Deactivate Stance : Outport  Port=3
  wires:
  Constant/1 -> Activate Swing/1
  Constant1/1 -> Reset/1
  Constant2/1 -> Deactivate Stance/1

== system Custom_Library/Signal Generator(Gen. 2)/Subsystem/If Action Subsystem1 ==
  Action Port : ActionPort
  Constant : Constant
  Constant1 : Constant  Value=0
  Constant2 : Constant  Value=0
  Activate Stance : Outport
  Reset : Outport  Port=2
  Deactivate Swing : Outport  Port=3
  wires:
  Constant/1 -> Activate Stance/1
  Constant1/1 -> Reset/1
  Constant2/1 -> Deactivate Swing/1

== system Custom_Library/Signal Generator(Gen. 2)/Subsystem/If Action Subsystem2 ==
  Action Port : ActionPort
  Constant1 : Constant
  Reset : Outport
  wires:
  Constant1/1 -> Reset/1

== system Custom_Library/Swing-Stance Pattern Generation/Swing-Stance Signal Generation/Enable Outputs ==
  X in : Inport
  Z in : Inport  Port=2
  Enable : Inport  Port=3
  Constant1 : Constant  Value=0
  Constant2 : Constant  Value=0
  Enable Outputs : Subsystem  TreatAsAtomicUnit=on
  Switch : Switch  Criteria=u2 > Threshold  SaturateOnIntegerOverflow=off  InputSameDT=off
  Switch1 : Switch  Criteria=u2 > Threshold  SaturateOnIntegerOverflow=off  InputSameDT=off
  X out : Outport  InitialOutput=0
  Z out : Outport  Port=2  InitialOutput=0
  wires:
  Switch1/1 -> Z out/1
  Z in/1 -> Switch1/1
  Constant2/1 -> Switch1/3
  Constant1/1 -> Switch/3
  X in/1 -> Switch/1
  Switch/1 -> X out/1
  Enable/1 -> Enable Outputs/Enable
  Enable Outputs/1(Enabled) -> Switch1/2, Switch/2

== system Custom_Library/Swing-Stance Pattern Generation/Swing-Stance Signal Generation/Trajectory Generation - Stance Phase (Adaptive PEP) ==
  Stance Frequency : Inport
  Reset : ResetPort  DisableCoverage=on
  Abs : Abs  SaturateOnIntegerOverflow=off
  Constant : Constant
  Constant1 : Constant  Value=AEP
  Constant2 : Constant  Value=AEP
  Constant3 : Constant  Value=PEP
  Constant4 : Constant  Value=0
  Integrator : Integrator
  Product1 : Product
  Product2 : Product
  Saturation : Saturate  UpperLimit=AEP  LowerLimit=PEP
  Subtract : Sum  Inputs=+-
  Subtract1 : Sum  Inputs=+-
  X : Outport
  Z : Outport  Port=2
  wires:
  Constant4/1 -> Z/1
  Saturation/1 -> X/1
  Product1/1 -> Product2/1
  Abs/1 -> Product1/2
  Subtract1/1 -> Abs/1
  Constant3/1 -> Subtract1/2
  Constant1/1 -> Subtract1/1
  Stance Frequency/1 -> Product1/1
  Integrator/1 -> Product2/2
  Product2/1 -> Subtract/2
  Subtract/1 -> Saturation/1
  Constant2/1 -> Subtract/1
  Constant/1 -> Integrator/1

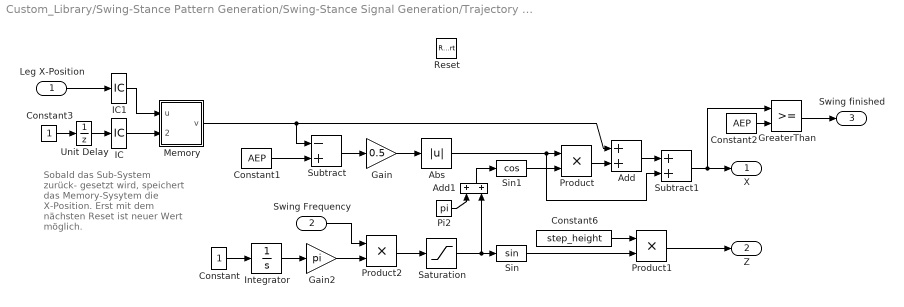
== system Custom_Library/Swing-Stance Pattern Generation/Swing-Stance Signal Generation/Trajectory Generation - Swing Phase (Adaptive PEP) ==
  note: Sobald das Sub-System zurück-
      | gesetzt wird, speichert das
      | Memory-Sysytem die X-Position.
      | Erst mit dem nächsten Reset ist
      | neuer Wert möglich.
  Leg X-Position : Inport
  Swing Frequency : Inport  Port=2
  Reset : ResetPort  DisableCoverage=on
  Abs : Abs  SaturateOnIntegerOverflow=off
  Add : Sum
  Add1 : Sum
  Constant : Constant
  Constant1 : Constant  Value=AEP
  Constant2 : Constant  Value=AEP
  Constant3 : Constant
  Constant6 : Constant  Value=step_height
  Gain : Gain  Gain=0.5
  Gain2 : Gain  Gain=pi
  GreaterThan : RelationalOperator  OutDataTypeStr=boolean  RndMeth=Simplest  InputSameDT=off
  IC : InitialCondition  Value=0
  IC1 : InitialCondition  Value=0
  Integrator : Integrator
  Memory : Subsystem
  Pi2 : Constant  Value=pi  OutDataTypeStr=Inherit: Inherit via back propagation
  Product : Product
  Product1 : Product
  Product2 : Product
  Saturation : Saturate  UpperLimit=pi  LowerLimit=0
  Sin : Trigonometry
  Sin1 : Trigonometry  Operator=cos
  Subtract : Sum  Inputs=-+
  Subtract1 : Sum
  Unit Delay : UnitDelay  SampleTime=-1  HasFrameUpgradeWarning=on
  X : Outport
  Z : Outport  Port=2
  Swing finished : Outport  Port=3
  wires:
  IC1/1 -> Memory/1(u)
  IC/1 -> Memory/2(Hold)
  Constant3/1 -> Unit Delay/1
  Unit Delay/1 -> IC/1
  Leg X-Position/1 -> IC1/1
  Swing Frequency/1 -> Product2/1
  Product2/1 -> Saturation/1
  Gain2/1 -> Product2/2
  Constant2/1 -> GreaterThan/2
  GreaterThan/1 -> Swing finished/1
  Constant/1 -> Integrator/1
  Integrator/1 -> Gain2/1
  Subtract1/1 -> GreaterThan/1, X/1
  Sin/1 -> Product1/2
  Gain/1 -> Abs/1
  Constant6/1 -> Product1/1
  Saturation/1 -> Sin/1, Add1/2
  Pi2/1 -> Add1/1
  Memory/1(v) -> Subtract/1, Add/1
  Product1/1 -> Z/1
  Constant1/1 -> Subtract/2
  Sin1/1 -> Product/2
  Add1/1 -> Sin1/1
  Add/1 -> Subtract1/1
  Subtract/1 -> Gain/1
  Abs/1 -> Product/1, Subtract1/2
  Product/1 -> Add/2

== system Custom_Library/Swing-Stance Pattern Generation/Swing-Stance Signal Generation/Enable Outputs/Enable Outputs ==
  Enable : EnablePort
  Constant : Constant
  IC : InitialCondition  Value=0
  Enabled : Outport  InitialOutput=0
  wires:
  Constant/1 -> IC/1
  IC/1 -> Enabled/1

== system Custom_Library/Swing-Stance Pattern Generation/Swing-Stance Signal Generation/Trajectory Generation - Swing Phase (Adaptive PEP)/Memory ==
  u : Inport
  Hold : Inport  Port=2
  Memory : Memory
  NOT : Logic  Operator=NOT  IconShape=distinctive  AllPortsSameDT=off  OutDataTypeStr=boolean
  Switch : Switch  Criteria=u2 > Threshold  SaturateOnIntegerOverflow=off  InputSameDT=off
  v : Outport
  wires:
  Memory/1 -> Switch/3
  u/1 -> Switch/1
  NOT/1 -> Switch/2
  Hold/1 -> NOT/1
  Switch/1 -> Memory/1, v/1
